simulink model "SDT_Control_Tuning"  (R2025b)
settings: Solver=VariableStepAuto  StartTime=0.0  StopTime=10.0  RelTol=1e-3
undefined symbols (not defined in the file or in its folder): boom, C_tile_force, C_tile_torque, CoM_variation_x, CoM_variation_y, CoM_variation_z, Container_x, Container_z, InvDyn, InvDynAug, J_B_B, J_C_C, J_P_P, J_T_T, K_tile_force, K_tile_torque, KIN, m_B, m_C, m_P, m_T, robot, Tile_z, unc_freq_boom, ureal, uss
libraries: SDTlibV1 x73, RCTblocks x39
(part 1 of 5)
settings Model: Creator=l.sekules  LastModifiedBy=l.sekules

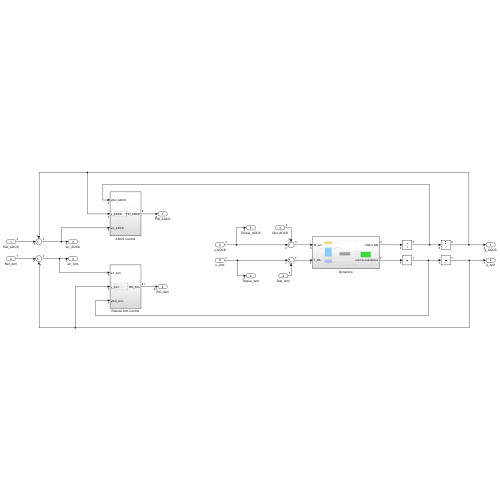
[thumbnail: Simulink's stored preview of the top-level diagram]
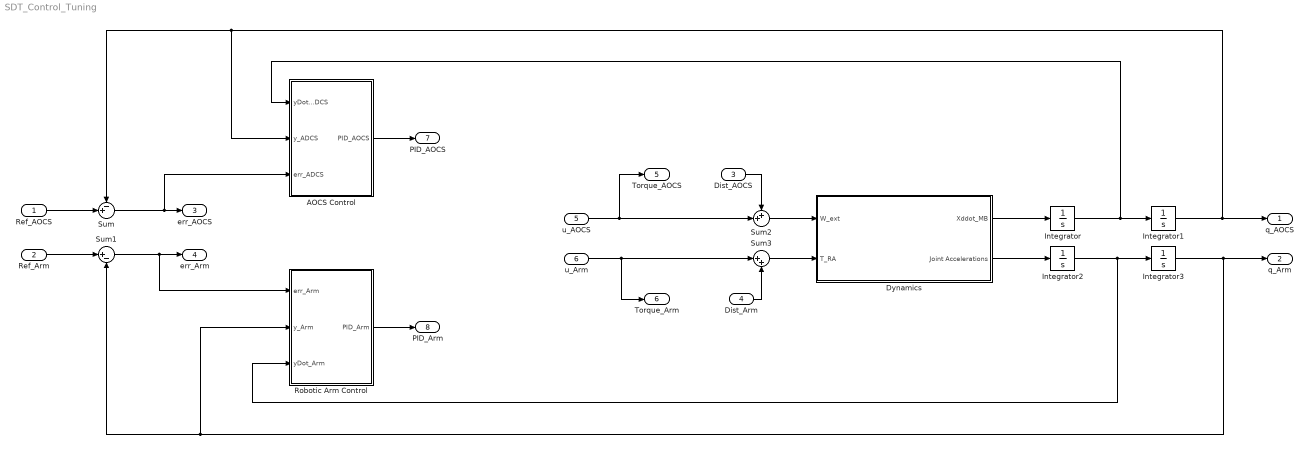
== system SDT_Control_Tuning ==
  Ref_AOCS : Inport  PortDimensions=3
  Ref_Arm : Inport  Port=2  PortDimensions=7
  Dist_AOCS : Inport  Port=3  PortDimensions=3
  Dist_Arm : Inport  Port=4  PortDimensions=7
  u_AOCS : Inport  Port=5  PortDimensions=3
  u_Arm : Inport  Port=6  PortDimensions=7
  AOCS Control : Subsystem
  Dynamics : Subsystem
  Integrator{,1..3} (4 alike) : Integrator
  Robotic Arm Control : Subsystem
  Sum : Sum  Inputs=-+|
  Sum1 : Sum  Inputs=|+-
  Sum2 : Sum  Inputs=++|
  Sum3 : Sum  Inputs=|++
  q_AOCS : Outport
  q_Arm : Outport  Port=2
  err_AOCS : Outport  Port=3
  err_Arm : Outport  Port=4
  Torque_AOCS : Outport  Port=5
  Torque_Arm : Outport  Port=6
  PID_AOCS : Outport  Port=7
  PID_Arm : Outport  Port=8
  wires:
  Integrator1/1 -> AOCS Control/2(y_ADCS), Sum/1, q_AOCS/1
  Integrator3/1 -> Robotic Arm Control/2(y_Arm), Sum1/2, q_Arm/1
  Sum/1 -> AOCS Control/3(err_ADCS), err_AOCS/1
  Sum1/1 -> Robotic Arm Control/1(err_Arm), err_Arm/1
  Ref_AOCS/1 -> Sum/2
  Ref_Arm/1 -> Sum1/1
  Integrator/1 -> AOCS Control/1(yDot_ADCS), Integrator1/1
  Integrator2/1 -> Robotic Arm Control/3(yDot_Arm), Integrator3/1
  AOCS Control/1(PID_AOCS) -> PID_AOCS/1
  Robotic Arm Control/1(PID_Arm) -> PID_Arm/1
  u_Arm/1 -> Torque_Arm/1, Sum3/1
  Dist_Arm/1 -> Sum3/2
  u_AOCS/1 -> Torque_AOCS/1, Sum2/2
  Dist_AOCS/1 -> Sum2/1
  Sum2/1 -> Dynamics/1(W_ext)
  Sum3/1 -> Dynamics/2(T_RA)
  Dynamics/1(Xddot_MB) -> Integrator/1
  Dynamics/2(Joint Accelerations) -> Integrator2/1

== system SDT_Control_Tuning/AOCS Control ==
  yDot_ADCS : Inport
  y_ADCS : Inport  Port=2
  err_ADCS : Inport  Port=3
  Integrator : Integrator
  Mux : Mux  Inputs=3
  PID_AOCS : Outport
  wires:
  err_ADCS/1 -> Integrator/1
  y_ADCS/1 -> Mux/1
  yDot_ADCS/1 -> Mux/3
  Mux/1 -> PID_AOCS/1
  Integrator/1 -> Mux/2

== system SDT_Control_Tuning/Dynamics ==
  W_ext : Inport
  T_RA : Inport  Port=2
  Demux : Demux  Outputs=3
  Demux1 : Demux  Outputs=2
  Flexible Bar : Subsystem
  Ground : Ground
  Main body : Subsystem  mask(Multi-port rigid body (18nx6n)){m=m_B, Ig=J_B_B, OG=[CoM_variation_x;CoM_variation_y;CoM_variation_z], n=4, OP1=[0;0;0], OP2=[0.35;0;2.5], OP3=[0;0;-2.5], OP4=[1.1;0;0.5], OP5=[0;0;0]}
      mask prompts: m "Mass (Kg)"; Ig "Inertia (at G, Kg m^2)"; OG "OG (3x1 vector, m)"; n "Number of ports"; OP1 "OP1 (3x1 vector, m)"; OP2 "OP2 (3x1 vector, m)"; OP3 "OP3 (3x1 vector, m)"; OP4 "OP4 (3x1 vector, m)"; OP5 "OP5 (3x1 vector,m)"
      mask help:
      | 18nx6n dynamic model of a rigid body at n given points (ports) between wrenches applied at the n points (input) and the motions vectors at these points (output).
      |
      | 0: the reference point
      | G: the center of mass
      | Pi (i=1:n): the n given connection points (n<6).
      |
      | All parameters are expressed in the body frame.
      | Each parameter can be an uncertain parameter declared with "ureal"
      mask init:
      | MultiPortRigidFreeBody
      mask Help: web('Docmultiportrigidbase.html','-browser','-browser')
      mask TypeOptions n: 1 | 2 | 3 | 4 | 5
      mask DialogControl ParameterGroupVar Prompt: Main parameters
      mask DialogControl port1 Prompt: Port #1
      mask DialogControl port2 Prompt: #2
      mask DialogControl port3 Prompt: #3
      mask DialogControl port4 Prompt: #4
      mask DialogControl port5 Prompt: #5
      mask Display:
      | disp('Multi-port\n rigid free body\n (18nx6n)')
      | for ii=1:n
      |     port_label('input', ii,['W_{./body,P',num2str(ii),'}'],'interpreter','tex')
      |     port_label('output',ii,['m_{P',num2str(ii),'}'],'interpreter','tex')
      | end
  Multi port rigid body : Subsystem  mask(Multi-port rigid body (18(n-1)+6]x[6(n-1)+18])){m=m_C, Ig=J_C_C, OG=[0;0;0], n=2, numinv=2, OP1=[Container_x/2;0;0], OP2=[0;0;-Container_z/2], OP3=[ureal('P3_y',1,'percent',10);0;0], OP4=[0;0;0], OP5=[0;0;0]}
      mask prompts: m "Mass (Kg)"; Ig "Inertia (at G, Kg m^2)"; OG "OG (3x1 vector, m)"; n "Number of ports"; numinv "The single parent port"; OP1 "OP1 (3x1 vector, m)"; OP2 "OP2 (3x1 vector, m)"; OP3 "OP3 (3x1 vector, m)"; OP4 "OP4 (3x1 vector, m)"; OP5 "OP5 (3x1 vector,m)"
      mask help:
      | [18(n-1)+6]x[6(n-1)+18] dynamic model of a rigid body at n given points (ports) between:
      | * the wrenches applied at the n-1 child ports and  the motion vector at a single parent port (inputs).
      | * the motions vectors at the  n-1 child ports and the wrench applied by the rigid body at the parent port (output)
      |
      | 0: the reference point
      | G: the center of mass
      | Pi (i=1:n): the n given connection points (n<6).
      |
      | All parameters are expressed in the body frame.
      | Each parameter can be an uncertain parameter declared with "ureal"
      |
      | The 6x18 channel associated to the single parent port can be any of the ports.
      mask init:
      | MultiPortRigidBodyAug
      mask Help: web('Docmultiportrigidbody.html','-browser','-browser')
      mask TypeOptions n: 1 | 2 | 3 | 4 | 5
      mask TypeOptions numinv: 1 | 2 | 3 | 4 | 5
      mask DialogControl ParameterGroupVar Prompt: Main parameters
      mask DialogControl port1 Prompt: Port #1
      mask DialogControl port2 Prompt: #2
      mask DialogControl port3 Prompt: #3
      mask DialogControl port4 Prompt: #4
      mask DialogControl port5 Prompt: #5
      mask Display:
      | disp('Multi-port\n rigid body\n [18(n-1)+6]x[6(n-1)+18]')
      | if n==1,
      |     if numinv==1,
      |         port_label('input', 1,'m_P')
      |         port_label('output',1,'Wbody/.,P')
      |     else
      |         port_label('input', 1,'W./body,P')
      |         port_label('output',1,'m_P')
      |     end
      | else
      |     for ii=1:n
      |         if numinv==ii,
      |             port_label('output',ii,['Wbody/.,P',num2str(ii)])
      |             port_label('input', ii,['m_P',num2str(ii)])
      |         else
      |             port_label('input', ii,['W./body,P',num2str(ii)])
      |             port_label('output',ii,['m_P',num2str(ii)])
      |         end
      |     end
      | end
  Mux : Mux  Inputs=2
  Robotic Arm : Subsystem
  Terminator : Terminator
  Terminator1 : Terminator
  Terminator2 : Terminator
  Tiles : Subsystem
  Xddot_MB : Outport
  Joint Accelerations : Outport  Port=2
  wires:
  Main body/4(m_P4) -> Robotic Arm/1(m_P1)
  Robotic Arm/2(Joint Accelerations) -> Joint Accelerations/1
  Demux/3 -> Terminator1/1
  Main body/2(m_P2) -> Multi port rigid body/2(in2)
  Tiles/3(W_EE) -> Robotic Arm/3(W_EE)
  Robotic Arm/1(W_P1) -> Main body/4(W_./body,P4)
  Multi port rigid body/1(out1) -> Tiles/1(m_Container)
  Robotic Arm/3(m_EE) -> Tiles/3(m_EE)
  Flexible Bar/2(m_Endpoint) -> Tiles/2(m_Endpoint)
  Tiles/2(W_Endpoint) -> Flexible Bar/2(W_Endpoint)
  Multi port rigid body/2(out2) -> Main body/2(W_./body,P2)
  Flexible Bar/1(W_body,P3) -> Main body/3(W_./body,P3)
  Main body/3(m_P3) -> Flexible Bar/1(m_P3)
  Main body/1(m_P1) -> Demux/1
  Demux/2 -> Terminator/1
  Tiles/1(W_Container) -> Multi port rigid body/1(in1)
  T_RA/1 -> Robotic Arm/2(T_RA)
  Demux/1 -> Demux1/1
  Demux1/2 -> Xddot_MB/1
  Demux1/1 -> Terminator2/1
  Mux/1 -> Main body/1(W_./body,P1)
  W_ext/1 -> Mux/2
  Ground/1 -> Mux/1

== system SDT_Control_Tuning/Robotic Arm Control ==
  err_Arm : Inport
  y_Arm : Inport  Port=2
  yDot_Arm : Inport  Port=3
  Integrator : Integrator
  Mux : Mux  Inputs=3
  PID_Arm : Outport
  wires:
  yDot_Arm/1 -> Mux/3
  y_Arm/1 -> Mux/1
  Integrator/1 -> Mux/2
  err_Arm/1 -> Integrator/1
  Mux/1 -> PID_Arm/1

== system SDT_Control_Tuning/Dynamics/Flexible Bar ==
  m_P3 : Inport
  W_Endpoint : Inport  Port=2
  " N ports Nastran (free) body" : Subsystem  mask(NINOP Model of a Nastran body){fbdf='boom', ff06='boom', P_gp=1, C_gp=11, nf=boom.n_modes, Xi=boom.damping_ratio, free=off, uw_var=unc_freq_boom, Nflex_w=boom.n_unc, uls_var=0, Nflex_LP=0, uev_var=0, Nflex_EV=0}
      mask prompts: fbdf "Name of the .bdf file (without extension)"; ff06 "Name of the .f06 file (without extension)"; P_gp "Node number corresponding to the point P (connection with parent body)"; C_gp "Node numbers corresponding to the points C (connections with child bodies)"; nf "Number of modes to be considered"; Xi "Common damping ratio"; free "Free body at P"; uw_var "uncertainties (%)"; Nflex_w "number of flexible modes (integer)"; uls_var "uncertainties (%)"; Nflex_LP "number of flexible modes (integer)"; uev_var "uncertainties (%)"; Nflex_EV "number of flexible modes (integer)"
      mask help:
      | NINOP (18n+6)x(6n+18) model of a flexible body at points C (connection point with the child  bodies) and point P (connection point with a parent body).
      | * 18nx6n transfer between the wrench applied to this body at the child points C  and motion vectors at these points
      | * 6x18 transfer between the motion vector at the "parent" point P  and the wrench applied by this body at this point
      | The model is expressed In the (inherit) body frame.
      |
      | Model is built from  the data provided by Patran/Nastran analysis output files.
      | Uncertainties can be added to the main parameters.
      |
      | RK: The last channel associated to parent port P can be inverted to free the body at the point P. In that case, 6 rigid modes (12 integrators) are added in the model to output the motion vector at the point P and the model becomes 18(n+1)x6(n+1).
      mask init:
      | n = length(C_gp);
      | NastranBodyNPortAugFree
      mask Help: web('DocNPortNastranBody.html','-browser','-browser')
      mask DialogControl Container2 Prompt: Main parameters
      mask DialogControl Container6 Prompt: Parametric uncertainties:
      mask DialogControl Container8 Prompt: Frequencies
      mask DialogControl Control18 Prompt: A common relative uncertainty (%) on the first flexible mode frequencies can be added (uncertainties can be changed later)
      mask DialogControl Control3 Prompt: The uncertain frequency is named: 'w_name_i' where:
      mask DialogControl Control4 Prompt: * 'name' is the current block name (reduced to its alphanumeric characters).
      mask DialogControl Control17 Prompt: * 'i' is the flexible mode number (increasing frequency order)
      mask DialogControl Container9 Prompt: Modal participation factors
      mask DialogControl Control20 Prompt: A common relative uncertainty (%) on the modal participation factors of the first flexible modes can be added (uncertainties can be changed later)
      mask DialogControl Control6 Prompt: The uncertain modal participation factor is named: 'LP_name_iXX' where:
      mask DialogControl Control7 Prompt: *  'name' is the current block name (reduced to its alphanumeric characters),
      mask DialogControl Control8 Prompt: * 'i' is the flexible mode number (increasing frequency order),
      mask DialogControl Control9 Prompt: * 'XX' = 'Tx', 'Ty', 'Tz', 'Rx', 'Ry', 'Rz'.
      mask DialogControl Container10 Prompt: Modal shapes
      mask DialogControl Control21 Prompt: A common relative uncertainty (%) on each eigen vector components at points C for the first flexible modes can be added (uncertainties can be changed later)
      mask DialogControl Control16 Prompt: WARNING: can generate very long process time !!
      mask DialogControl Control11 Prompt: The uncertain component is named: "EV_name_Cj_iXX' where:
      mask DialogControl Control12 Prompt: * 'name' is the current block name (reduced to its alphanumeric characters).
      mask DialogControl Control13 Prompt: * 'j' is the point C number,
      mask DialogControl Control14 Prompt: * 'i' is the flexible mode number (increasing frequency order),
      mask DialogControl Control15 Prompt: * 'XX' = 'Tx', 'Ty', 'Tz', 'Rx', 'Ry', 'Rz'.
      mask Display:
      | if free
      |     disp('NINOP (free)\n Nastran body\n 18(n+1)x6(n+1)')
      | else
      |     disp('NINOP (free)\n Nastran body\n (18n+6)x(6n+18)')
      | end
      | 
      | for ii=1:n
      |         port_label('input', ii,['W./body,C',num2str(ii)])
      |         port_label('output',ii,['m_C',num2str(ii)])
      | end
      | 
      | if free
      |     port_label('input', n+1,'W./body,P')
      |     port_label('output',n+1,'m_P')
      | else
      |     port_label('input', n+1,'m_P')
      |     port_label('output',n+1,'Wbody/.,P')
      | end
  18x18 DCM : SDTlibV1/3//6//18 DCM/18x18 DCM  rot=[0 0 1;0 1 0; -1 0 0]'  transp=off
      settings: SourceProductName=SDTlib
  18x18 DCM1 : SDTlibV1/3//6//18 DCM/18x18 DCM  rot=[0 -1 0; 1 0 0; 0 0 1]'  transp=off
      settings: SourceProductName=SDTlib
  18x18 DCM2 : SDTlibV1/3//6//18 DCM/18x18 DCM  rot=[0 0 1;0 1 0; -1 0 0]  transp=off
      settings: SourceProductName=SDTlib
  6x6 DCM : SDTlibV1/3//6//18 DCM/6x6 DCM  rot=[0 0 1;0 1 0; -1 0 0]  transp=off
      settings: SourceProductName=SDTlib
  6x6 DCM1 : SDTlibV1/3//6//18 DCM/6x6 DCM  rot=[0 -1 0; 1 0 0; 0 0 1]  transp=off
      settings: SourceProductName=SDTlib
  6x6 DCM2 : SDTlibV1/3//6//18 DCM/6x6 DCM  rot=[0 0 1;0 1 0; -1 0 0]'  transp=off
      settings: SourceProductName=SDTlib
  Multi port rigid body1 : Subsystem  mask(Multi-port rigid body (18(n-1)+6]x[6(n-1)+18])){m=m_P, Ig=J_P_P, OG=[0;0;0], n=2, numinv=1, OP1=[0;0;0.2], OP2=[0.1;0;-0.1], OP3=[ureal('P3_y',1,'percent',10);0;0], OP4=[0;0;0], OP5=[0;0;0]}
      mask prompts: m "Mass (Kg)"; Ig "Inertia (at G, Kg m^2)"; OG "OG (3x1 vector, m)"; n "Number of ports"; numinv "The single parent port"; OP1 "OP1 (3x1 vector, m)"; OP2 "OP2 (3x1 vector, m)"; OP3 "OP3 (3x1 vector, m)"; OP4 "OP4 (3x1 vector, m)"; OP5 "OP5 (3x1 vector,m)"
      mask help:
      | [18(n-1)+6]x[6(n-1)+18] dynamic model of a rigid body at n given points (ports) between:
      | * the wrenches applied at the n-1 child ports and  the motion vector at a single parent port (inputs).
      | * the motions vectors at the  n-1 child ports and the wrench applied by the rigid body at the parent port (output)
      |
      | 0: the reference point
      | G: the center of mass
      | Pi (i=1:n): the n given connection points (n<6).
      |
      | All parameters are expressed in the body frame.
      | Each parameter can be an uncertain parameter declared with "ureal"
      |
      | The 6x18 channel associated to the single parent port can be any of the ports.
      mask init:
      | MultiPortRigidBodyAug
      mask Help: web('Docmultiportrigidbody.html','-browser','-browser')
      mask TypeOptions n: 1 | 2 | 3 | 4 | 5
      mask TypeOptions numinv: 1 | 2 | 3 | 4 | 5
      mask DialogControl ParameterGroupVar Prompt: Main parameters
      mask DialogControl port1 Prompt: Port #1
      mask DialogControl port2 Prompt: #2
      mask DialogControl port3 Prompt: #3
      mask DialogControl port4 Prompt: #4
      mask DialogControl port5 Prompt: #5
      mask Display:
      | disp('Multi-port\n rigid body\n [18(n-1)+6]x[6(n-1)+18]')
      | if n==1,
      |     if numinv==1,
      |         port_label('input', 1,'m_P')
      |         port_label('output',1,'Wbody/.,P')
      |     else
      |         port_label('input', 1,'W./body,P')
      |         port_label('output',1,'m_P')
      |     end
      | else
      |     for ii=1:n
      |         if numinv==ii,
      |             port_label('output',ii,['Wbody/.,P',num2str(ii)])
      |             port_label('input', ii,['m_P',num2str(ii)])
      |         else
      |             port_label('input', ii,['W./body,P',num2str(ii)])
      |             port_label('output',ii,['m_P',num2str(ii)])
      |         end
      |     end
      | end
  Multi port rigid body2 : Subsystem  mask(Multi-port rigid body (18(n-1)+6]x[6(n-1)+18])){m=m_P, Ig=J_P_P, OG=[0;0;0], n=2, numinv=1, OP1=[-0.1 0 -0.1], OP2=[0 0 0.2], OP3=[ureal('P3_y',1,'percent',10);0;0], OP4=[0;0;0], OP5=[0;0;0]}
      mask prompts: m "Mass (Kg)"; Ig "Inertia (at G, Kg m^2)"; OG "OG (3x1 vector, m)"; n "Number of ports"; numinv "The single parent port"; OP1 "OP1 (3x1 vector, m)"; OP2 "OP2 (3x1 vector, m)"; OP3 "OP3 (3x1 vector, m)"; OP4 "OP4 (3x1 vector, m)"; OP5 "OP5 (3x1 vector,m)"
      mask help:
      | [18(n-1)+6]x[6(n-1)+18] dynamic model of a rigid body at n given points (ports) between:
      | * the wrenches applied at the n-1 child ports and  the motion vector at a single parent port (inputs).
      | * the motions vectors at the  n-1 child ports and the wrench applied by the rigid body at the parent port (output)
      |
      | 0: the reference point
      | G: the center of mass
      | Pi (i=1:n): the n given connection points (n<6).
      |
      | All parameters are expressed in the body frame.
      | Each parameter can be an uncertain parameter declared with "ureal"
      |
      | The 6x18 channel associated to the single parent port can be any of the ports.
      mask init:
      | MultiPortRigidBodyAug
      mask Help: web('Docmultiportrigidbody.html','-browser','-browser')
      mask TypeOptions n: 1 | 2 | 3 | 4 | 5
      mask TypeOptions numinv: 1 | 2 | 3 | 4 | 5
      mask DialogControl ParameterGroupVar Prompt: Main parameters
      mask DialogControl port1 Prompt: Port #1
      mask DialogControl port2 Prompt: #2
      mask DialogControl port3 Prompt: #3
      mask DialogControl port4 Prompt: #4
      mask DialogControl port5 Prompt: #5
      mask Display:
      | disp('Multi-port\n rigid body\n [18(n-1)+6]x[6(n-1)+18]')
      | if n==1,
      |     if numinv==1,
      |         port_label('input', 1,'m_P')
      |         port_label('output',1,'Wbody/.,P')
      |     else
      |         port_label('input', 1,'W./body,P')
      |         port_label('output',1,'m_P')
      |     end
      | else
      |     for ii=1:n
      |         if numinv==ii,
      |             port_label('output',ii,['Wbody/.,P',num2str(ii)])
      |             port_label('input', ii,['m_P',num2str(ii)])
      |         else
      |             port_label('input', ii,['W./body,P',num2str(ii)])
      |             port_label('output',ii,['m_P',num2str(ii)])
      |         end
      |     end
      | end
  W_body,P3 : Outport
  m_Endpoint : Outport  Port=2
  wires:
  " N ports Nastran (free) body"/2(out2) -> 6x6 DCM/1
  " N ports Nastran (free) body"/1(out1) -> 18x18 DCM2/1
  Multi port rigid body1/2(out2) -> 18x18 DCM/1
  6x6 DCM2/1 -> " N ports Nastran (free) body"/1(in1)
  18x18 DCM2/1 -> Multi port rigid body2/1(in1)
  6x6 DCM/1 -> Multi port rigid body1/2(in2)
  18x18 DCM/1 -> " N ports Nastran (free) body"/2(in2)
  Multi port rigid body2/1(out1) -> 6x6 DCM2/1
  6x6 DCM1/1 -> Multi port rigid body2/2(in2)
  Multi port rigid body2/2(out2) -> 18x18 DCM1/1
  Multi port rigid body1/1(out1) -> W_body,P3/1
  m_P3/1 -> Multi port rigid body1/1(in1)
  18x18 DCM1/1 -> m_Endpoint/1
  W_Endpoint/1 -> 6x6 DCM1/1

== system SDT_Control_Tuning/Dynamics/Main body ==
  W_./body,P1 : Inport  PortDimensions=6
  W_./body,P2 : Inport  Port=2  PortDimensions=6
  W_./body,P3 : Inport  Port=3  PortDimensions=6
  W_./body,P4 : Inport  Port=4  PortDimensions=6
  Demux : Demux  Outputs=[18 18 18 18]
  Gain : RCTblocks/Uncertain State Space  Tag=USS  USystem=uss(InvDyn)  UValue=[]  X0=[]  uX0=[]
  Mux : Mux  Inputs=[6 6 6 6]
  m_P1 : Outport
  m_P2 : Outport  Port=2
  m_P3 : Outport  Port=3
  m_P4 : Outport  Port=4
  wires:
  Mux/1 -> Gain/1
  Gain/1 -> Demux/1
  W_./body,P1/1 -> Mux/1
  Demux/1 -> m_P1/1
  W_./body,P2/1 -> Mux/2
  Demux/2 -> m_P2/1
  W_./body,P3/1 -> Mux/3
  Demux/3 -> m_P3/1
  W_./body,P4/1 -> Mux/4
  Demux/4 -> m_P4/1

== system SDT_Control_Tuning/Dynamics/Multi port rigid body ==
  in1 : Inport  PortDimensions=6
  in2 : Inport  Port=2  PortDimensions=18
  Demux : Demux  Outputs=[ 18 6]
  Gain : RCTblocks/Uncertain State Space  Tag=USS  USystem=uss(InvDynAug)  UValue=[]  X0=[]  uX0=[]
  Mux : Mux  Inputs=[ 6 18]
  out1 : Outport
  out2 : Outport  Port=2
  wires:
  Mux/1 -> Gain/1
  Gain/1 -> Demux/1
  in1/1 -> Mux/1
  Demux/1 -> out1/1
  in2/1 -> Mux/2
  Demux/2 -> out2/1

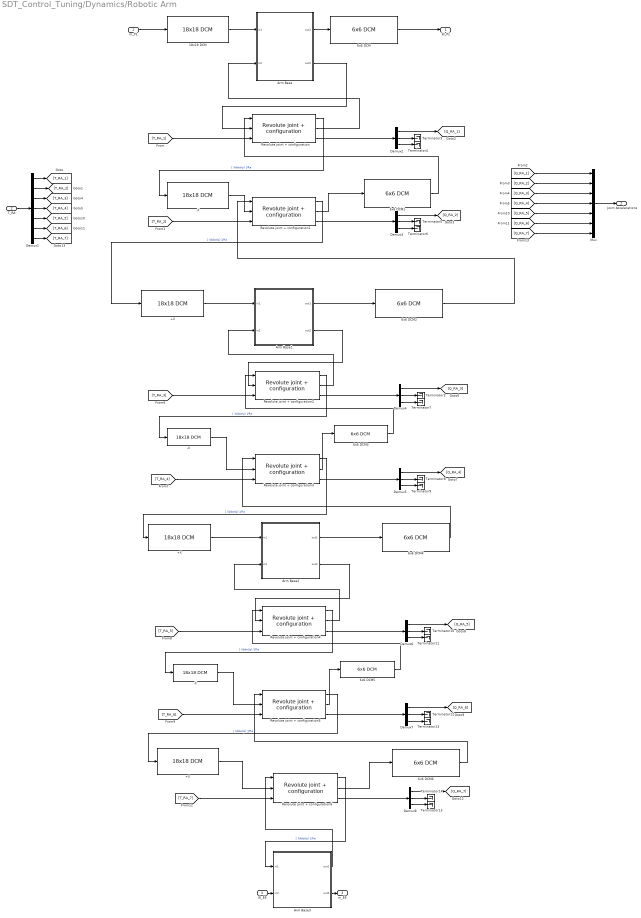
== system SDT_Control_Tuning/Dynamics/Robotic Arm ==
  m_P1 : Inport
  T_RA : Inport  Port=2
  W_EE : Inport  Port=3
  +X : SDTlibV1/3//6//18 DCM/18x18 DCM  rot=[1 0 0; 0 0 1; 0 -1 0]  transp=off
      settings: SourceProductName=SDTlib
  "+X " : SDTlibV1/3//6//18 DCM/18x18 DCM  rot=[1 0 0; 0 0 1; 0 -1 0]  transp=off
      settings: SourceProductName=SDTlib
  "+X  " : SDTlibV1/3//6//18 DCM/18x18 DCM  rot=[1 0 0; 0 0 1; 0 -1 0]  transp=off
      settings: SourceProductName=SDTlib
  -X : SDTlibV1/3//6//18 DCM/18x18 DCM  rot=[1 0 0; 0 0 1; 0 -1 0]  transp=on
      settings: SourceProductName=SDTlib
  "-X " : SDTlibV1/3//6//18 DCM/18x18 DCM  rot=[1 0 0; 0 0 1; 0 -1 0]  transp=on
      settings: SourceProductName=SDTlib
  "-X   " : SDTlibV1/3//6//18 DCM/18x18 DCM  rot=[1 0 0; 0 0 1; 0 -1 0]  transp=on
      settings: SourceProductName=SDTlib
  18x18 DCM : SDTlibV1/3//6//18 DCM/18x18 DCM  rot=[0 0 1;0 1 0; -1 0 0]'  transp=off
      settings: SourceProductName=SDTlib
  6x6 DCM : SDTlibV1/3//6//18 DCM/6x6 DCM  rot=[0 0 1;0 1 0; -1 0 0]  transp=off
      settings: SourceProductName=SDTlib
  6x6 DCM1 : SDTlibV1/3//6//18 DCM/6x6 DCM  rot=[1 0 0; 0 0 1; 0 -1 0]  transp=off
      settings: SourceProductName=SDTlib
  6x6 DCM2 : SDTlibV1/3//6//18 DCM/6x6 DCM  rot=[1 0 0; 0 0 1; 0 -1 0]  transp=on
      settings: SourceProductName=SDTlib
  6x6 DCM3 : SDTlibV1/3//6//18 DCM/6x6 DCM  rot=[1 0 0; 0 0 1; 0 -1 0]  transp=off
      settings: SourceProductName=SDTlib
  6x6 DCM4 : SDTlibV1/3//6//18 DCM/6x6 DCM  rot=[1 0 0; 0 0 1; 0 -1 0]  transp=on
      settings: SourceProductName=SDTlib
  6x6 DCM5 : SDTlibV1/3//6//18 DCM/6x6 DCM  rot=[1 0 0; 0 0 1; 0 -1 0]  transp=off
      settings: SourceProductName=SDTlib
  6x6 DCM6 : SDTlibV1/3//6//18 DCM/6x6 DCM  rot=[1 0 0; 0 0 1; 0 -1 0]  transp=on
      settings: SourceProductName=SDTlib
  Arm Base : Subsystem  mask(Multi-port rigid body (18(n-1)+6]x[6(n-1)+18])){m=robot.linkMass{1,1}, Ig=robot.linkInertia{1,1}, OG=[0;0;0], n=2, numinv=1, OP1=[0;0;-robot.linkLength(1)/2], OP2=[0;0;robot.linkLength(1)/2], OP3=[ureal('P3_y',1,'percent',10);0;0], OP4=[0;0;0], OP5=[0;0;0]}
      mask prompts: m "Mass (Kg)"; Ig "Inertia (at G, Kg m^2)"; OG "OG (3x1 vector, m)"; n "Number of ports"; numinv "The single parent port"; OP1 "OP1 (3x1 vector, m)"; OP2 "OP2 (3x1 vector, m)"; OP3 "OP3 (3x1 vector, m)"; OP4 "OP4 (3x1 vector, m)"; OP5 "OP5 (3x1 vector,m)"
      mask help:
      | [18(n-1)+6]x[6(n-1)+18] dynamic model of a rigid body at n given points (ports) between:
      | * the wrenches applied at the n-1 child ports and  the motion vector at a single parent port (inputs).
      | * the motions vectors at the  n-1 child ports and the wrench applied by the rigid body at the parent port (output)
      |
      | 0: the reference point
      | G: the center of mass
      | Pi (i=1:n): the n given connection points (n<6).
      |
      | All parameters are expressed in the body frame.
      | Each parameter can be an uncertain parameter declared with "ureal"
      |
      | The 6x18 channel associated to the single parent port can be any of the ports.
      mask init:
      | MultiPortRigidBodyAug
      mask Help: web('Docmultiportrigidbody.html','-browser','-browser')
      mask TypeOptions n: 1 | 2 | 3 | 4 | 5
      mask TypeOptions numinv: 1 | 2 | 3 | 4 | 5
      mask DialogControl ParameterGroupVar Prompt: Main parameters
      mask DialogControl port1 Prompt: Port #1
      mask DialogControl port2 Prompt: #2
      mask DialogControl port3 Prompt: #3
      mask DialogControl port4 Prompt: #4
      mask DialogControl port5 Prompt: #5
      mask Display:
      | disp('Multi-port\n rigid body\n [18(n-1)+6]x[6(n-1)+18]')
      | if n==1,
      |     if numinv==1,
      |         port_label('input', 1,'m_P')
      |         port_label('output',1,'Wbody/.,P')
      |     else
      |         port_label('input', 1,'W./body,P')
      |         port_label('output',1,'m_P')
      |     end
      | else
      |     for ii=1:n
      |         if numinv==ii,
      |             port_label('output',ii,['Wbody/.,P',num2str(ii)])
      |             port_label('input', ii,['m_P',num2str(ii)])
      |         else
      |             port_label('input', ii,['W./body,P',num2str(ii)])
      |             port_label('output',ii,['m_P',num2str(ii)])
      |         end
      |     end
      | end
  Arm Base1 : Subsystem  mask(Multi-port rigid body (18(n-1)+6]x[6(n-1)+18])){m=robot.linkMass{1,2}, Ig=robot.linkInertia{1,2}, OG=[0;0;0], n=2, numinv=1, OP1=[0;0;-robot.linkLength(2)/2], OP2=[0;0;robot.linkLength(2)/2], OP3=[ureal('P3_y',1,'percent',10);0;0], OP4=[0;0;0], OP5=[0;0;0]}
      mask prompts: m "Mass (Kg)"; Ig "Inertia (at G, Kg m^2)"; OG "OG (3x1 vector, m)"; n "Number of ports"; numinv "The single parent port"; OP1 "OP1 (3x1 vector, m)"; OP2 "OP2 (3x1 vector, m)"; OP3 "OP3 (3x1 vector, m)"; OP4 "OP4 (3x1 vector, m)"; OP5 "OP5 (3x1 vector,m)"
      mask help:
      | [18(n-1)+6]x[6(n-1)+18] dynamic model of a rigid body at n given points (ports) between:
      | * the wrenches applied at the n-1 child ports and  the motion vector at a single parent port (inputs).
      | * the motions vectors at the  n-1 child ports and the wrench applied by the rigid body at the parent port (output)
      |
      | 0: the reference point
      | G: the center of mass
      | Pi (i=1:n): the n given connection points (n<6).
      |
      | All parameters are expressed in the body frame.
      | Each parameter can be an uncertain parameter declared with "ureal"
      |
      | The 6x18 channel associated to the single parent port can be any of the ports.
      mask init:
      | MultiPortRigidBodyAug
      mask Help: web('Docmultiportrigidbody.html','-browser','-browser')
      mask TypeOptions n: 1 | 2 | 3 | 4 | 5
      mask TypeOptions numinv: 1 | 2 | 3 | 4 | 5
      mask DialogControl ParameterGroupVar Prompt: Main parameters
      mask DialogControl port1 Prompt: Port #1
      mask DialogControl port2 Prompt: #2
      mask DialogControl port3 Prompt: #3
      mask DialogControl port4 Prompt: #4
      mask DialogControl port5 Prompt: #5
      mask Display:
      | disp('Multi-port\n rigid body\n [18(n-1)+6]x[6(n-1)+18]')
      | if n==1,
      |     if numinv==1,
      |         port_label('input', 1,'m_P')
      |         port_label('output',1,'Wbody/.,P')
      |     else
      |         port_label('input', 1,'W./body,P')
      |         port_label('output',1,'m_P')
      |     end
      | else
      |     for ii=1:n
      |         if numinv==ii,
      |             port_label('output',ii,['Wbody/.,P',num2str(ii)])
      |             port_label('input', ii,['m_P',num2str(ii)])
      |         else
      |             port_label('input', ii,['W./body,P',num2str(ii)])
      |             port_label('output',ii,['m_P',num2str(ii)])
      |         end
      |     end
      | end
  Arm Base2 : Subsystem  mask(Multi-port rigid body (18(n-1)+6]x[6(n-1)+18])){m=robot.linkMass{1,3}, Ig=robot.linkInertia{1,3}, OG=[0;0;0], n=2, numinv=1, OP1=[0;0;-robot.linkLength(3)/2], OP2=[0;0;robot.linkLength(3)/2], OP3=[ureal('P3_y',1,'percent',10);0;0], OP4=[0;0;0], OP5=[0;0;0]}
      mask prompts: m "Mass (Kg)"; Ig "Inertia (at G, Kg m^2)"; OG "OG (3x1 vector, m)"; n "Number of ports"; numinv "The single parent port"; OP1 "OP1 (3x1 vector, m)"; OP2 "OP2 (3x1 vector, m)"; OP3 "OP3 (3x1 vector, m)"; OP4 "OP4 (3x1 vector, m)"; OP5 "OP5 (3x1 vector,m)"
      mask help:
      | [18(n-1)+6]x[6(n-1)+18] dynamic model of a rigid body at n given points (ports) between:
      | * the wrenches applied at the n-1 child ports and  the motion vector at a single parent port (inputs).
      | * the motions vectors at the  n-1 child ports and the wrench applied by the rigid body at the parent port (output)
      |
      | 0: the reference point
      | G: the center of mass
      | Pi (i=1:n): the n given connection points (n<6).
      |
      | All parameters are expressed in the body frame.
      | Each parameter can be an uncertain parameter declared with "ureal"
      |
      | The 6x18 channel associated to the single parent port can be any of the ports.
      mask init:
      | MultiPortRigidBodyAug
      mask Help: web('Docmultiportrigidbody.html','-browser','-browser')
      mask TypeOptions n: 1 | 2 | 3 | 4 | 5
      mask TypeOptions numinv: 1 | 2 | 3 | 4 | 5
      mask DialogControl ParameterGroupVar Prompt: Main parameters
      mask DialogControl port1 Prompt: Port #1
      mask DialogControl port2 Prompt: #2
      mask DialogControl port3 Prompt: #3
      mask DialogControl port4 Prompt: #4
      mask DialogControl port5 Prompt: #5
      mask Display:
      | disp('Multi-port\n rigid body\n [18(n-1)+6]x[6(n-1)+18]')
      | if n==1,
      |     if numinv==1,
      |         port_label('input', 1,'m_P')
      |         port_label('output',1,'Wbody/.,P')
      |     else
      |         port_label('input', 1,'W./body,P')
      |         port_label('output',1,'m_P')
      |     end
      | else
      |     for ii=1:n
      |         if numinv==ii,
      |             port_label('output',ii,['Wbody/.,P',num2str(ii)])
      |             port_label('input', ii,['m_P',num2str(ii)])
      |         else
      |             port_label('input', ii,['W./body,P',num2str(ii)])
      |             port_label('output',ii,['m_P',num2str(ii)])
      |         end
      |     end
      | end
  Arm Base3 : Subsystem  mask(Multi-port rigid body (18(n-1)+6]x[6(n-1)+18])){m=robot.linkMass{1,4}, Ig=robot.linkInertia{1,4}, OG=[0;0;0], n=2, numinv=1, OP1=[0;0;-robot.linkLength(4)/2], OP2=[0;0;robot.linkLength(4)/2], OP3=[ureal('P3_y',1,'percent',10);0;0], OP4=[0;0;0], OP5=[0;0;0]}
      mask prompts: m "Mass (Kg)"; Ig "Inertia (at G, Kg m^2)"; OG "OG (3x1 vector, m)"; n "Number of ports"; numinv "The single parent port"; OP1 "OP1 (3x1 vector, m)"; OP2 "OP2 (3x1 vector, m)"; OP3 "OP3 (3x1 vector, m)"; OP4 "OP4 (3x1 vector, m)"; OP5 "OP5 (3x1 vector,m)"
      mask help:
      | [18(n-1)+6]x[6(n-1)+18] dynamic model of a rigid body at n given points (ports) between:
      | * the wrenches applied at the n-1 child ports and  the motion vector at a single parent port (inputs).
      | * the motions vectors at the  n-1 child ports and the wrench applied by the rigid body at the parent port (output)
      |
      | 0: the reference point
      | G: the center of mass
      | Pi (i=1:n): the n given connection points (n<6).
      |
      | All parameters are expressed in the body frame.
      | Each parameter can be an uncertain parameter declared with "ureal"
      |
      | The 6x18 channel associated to the single parent port can be any of the ports.
      mask init:
      | MultiPortRigidBodyAug
      mask Help: web('Docmultiportrigidbody.html','-browser','-browser')
      mask TypeOptions n: 1 | 2 | 3 | 4 | 5
      mask TypeOptions numinv: 1 | 2 | 3 | 4 | 5
      mask DialogControl ParameterGroupVar Prompt: Main parameters
      mask DialogControl port1 Prompt: Port #1
      mask DialogControl port2 Prompt: #2
      mask DialogControl port3 Prompt: #3
      mask DialogControl port4 Prompt: #4
      mask DialogControl port5 Prompt: #5
      mask Display:
      | disp('Multi-port\n rigid body\n [18(n-1)+6]x[6(n-1)+18]')
      | if n==1,
      |     if numinv==1,
      |         port_label('input', 1,'m_P')
      |         port_label('output',1,'Wbody/.,P')
      |     else
      |         port_label('input', 1,'W./body,P')
      |         port_label('output',1,'m_P')
      |     end
      | else
      |     for ii=1:n
      |         if numinv==ii,
      |             port_label('output',ii,['Wbody/.,P',num2str(ii)])
      |             port_label('input', ii,['m_P',num2str(ii)])
      |         else
      |             port_label('input', ii,['W./body,P',num2str(ii)])
      |             port_label('output',ii,['m_P',num2str(ii)])
      |         end
      |     end
      | end
  Demux1 : Demux  Outputs=7
  Demux{2..8} (7 alike) : Demux  Outputs=3
  Mux : Mux  Inputs=7
  Revolute joint + configuration : SDTlibV1/6 dof mechanisms/Revolute joint + configuration  ra=[0;0;1]  Jr=1  theta=robot.config{1}
      settings: SourceProductName=SDTlib
  Revolute joint + configuration1 : SDTlibV1/6 dof mechanisms/Revolute joint + configuration  ra=[0;0;1]  Jr=1  theta=robot.config{2}
      settings: SourceProductName=SDTlib
  Revolute joint + configuration2 : SDTlibV1/6 dof mechanisms/Revolute joint + configuration  ra=[0;0;1]  Jr=1  theta=robot.config{3}
      settings: SourceProductName=SDTlib
  Revolute joint + configuration3 : SDTlibV1/6 dof mechanisms/Revolute joint + configuration  ra=[0;0;1]  Jr=1  theta=robot.config{4}
      settings: SourceProductName=SDTlib
  Revolute joint + configuration4 : SDTlibV1/6 dof mechanisms/Revolute joint + configuration  ra=[0;0;1]  Jr=1  theta=robot.config{5}
      settings: SourceProductName=SDTlib
  Revolute joint + configuration5 : SDTlibV1/6 dof mechanisms/Revolute joint + configuration  ra=[0;0;1]  Jr=1  theta=robot.config{6}
      settings: SourceProductName=SDTlib
  Revolute joint + configuration6 : SDTlibV1/6 dof mechanisms/Revolute joint + configuration  ra=[0;0;1]  Jr=1  theta=robot.config{7}
      settings: SourceProductName=SDTlib
  Terminator{2..15} (14 alike) : Terminator
  W_P1 : Outport
  Joint Accelerations : Outport  Port=2
  m_EE : Outport  Port=3
  wires:
  Demux4/3 -> Terminator7/1
  6x6 DCM3/1 -> Revolute joint + configuration2/1
  Demux6/1 -> [Q_RA_5]
  Demux8/1 -> [Q_RA_7]
  [Q_RA_3] -> Mux/3
  Demux7/2 -> Terminator12/1
  Revolute joint + configuration/2 -> Arm Base/2(in2)
  Demux3/1 -> [Q_RA_2]
  [T_RA_3] -> Revolute joint + configuration2/3
  Arm Base/1(out1) -> 6x6 DCM/1
  Revolute joint + configuration4/2 -> Arm Base2/2(in2)
  Arm Base3/1(out1) -> Revolute joint + configuration6/1
  Revolute joint + configuration/1 -> "-X "/1  "[ Xddot(p) ]/Ra"
  [T_RA_7] -> Revolute joint + configuration6/3
  Arm Base/2(out2) -> Revolute joint + configuration/2
  [T_RA_4] -> Revolute joint + configuration3/3
  Revolute joint + configuration5/3 -> Demux7/1
  Demux8/2 -> Terminator14/1
  Revolute joint + configuration4/3 -> Demux6/1
  Demux2/2 -> Terminator3/1
  [T_RA_5] -> Revolute joint + configuration4/3
  "+X  "/1 -> Revolute joint + configuration6/2
  [T_RA_1] -> Revolute joint + configuration/3
  Demux7/3 -> Terminator13/1
  Demux3/2 -> Terminator5/1
  Demux1/4 -> [T_RA_4]
  Revolute joint + configuration2/1 -> -X/1  "[ Xddot(p) ]/Ra"
  W_EE/1 -> Arm Base3/2(in2)
  Arm Base1/2(out2) -> Revolute joint + configuration2/2
  T_RA/1 -> Demux1/1
  Revolute joint + configuration2/3 -> Demux4/1
  Revolute joint + configuration/3 -> Demux2/1
  Demux7/1 -> [Q_RA_6]
  [Q_RA_4] -> Mux/4
  Demux1/2 -> [T_RA_2]
  Demux1/3 -> [T_RA_3]
  Demux6/2 -> Terminator10/1
  Demux6/3 -> Terminator11/1
  [Q_RA_5] -> Mux/5
  18x18 DCM/1 -> Arm Base/1(in1)
  "-X   "/1 -> Revolute joint + configuration5/2
  "-X "/1 -> Revolute joint + configuration1/2
  Demux3/3 -> Terminator6/1
  6x6 DCM5/1 -> Revolute joint + configuration4/1
  Arm Base2/1(out1) -> 6x6 DCM4/1
  Demux2/3 -> Terminator4/1
  Revolute joint + configuration4/1 -> "-X   "/1  "[ Xddot(p) ]/Ra"
  Revolute joint + configuration6/1 -> Arm Base3/1(in1)  "[ Xddot(p) ]/Ra"
  Demux4/2 -> Terminator2/1
  Revolute joint + configuration1/2 -> 6x6 DCM1/1
  [T_RA_6] -> Revolute joint + configuration5/3
  Revolute joint + configuration3/1 -> "+X "/1  "[ Xddot(p) ]/Ra"
  Demux5/1 -> [Q_RA_4]
  [T_RA_2] -> Revolute joint + configuration1/3
  [Q_RA_2] -> Mux/2
  "+X "/1 -> Arm Base2/1(in1)
  Mux/1 -> Joint Accelerations/1
  Demux4/1 -> [Q_RA_3]
  6x6 DCM1/1 -> Revolute joint + configuration/1
  Demux5/2 -> Terminator8/1
  +X/1 -> Arm Base1/1(in1)
  Revolute joint + configuration1/3 -> Demux3/1
  Revolute joint + configuration3/2 -> 6x6 DCM3/1
  -X/1 -> Revolute joint + configuration3/2
  Revolute joint + configuration2/2 -> Arm Base1/2(in2)
  6x6 DCM6/1 -> Revolute joint + configuration5/1
  Demux2/1 -> [Q_RA_1]
  Revolute joint + configuration6/3 -> Demux8/1
  Demux5/3 -> Terminator9/1
  [Q_RA_7] -> Mux/7
  [Q_RA_6] -> Mux/6
  Arm Base1/1(out1) -> 6x6 DCM2/1
  6x6 DCM4/1 -> Revolute joint + configuration3/1
  [Q_RA_1] -> Mux/1
  Revolute joint + configuration1/1 -> +X/1  "[ Xddot(p) ]/Ra"
  Revolute joint + configuration3/3 -> Demux5/1
  6x6 DCM2/1 -> Revolute joint + configuration1/1
  Demux1/1 -> [T_RA_1]
  Demux8/3 -> Terminator15/1
  Revolute joint + configuration6/2 -> 6x6 DCM6/1
  Arm Base2/2(out2) -> Revolute joint + configuration4/2
  Revolute joint + configuration5/2 -> 6x6 DCM5/1
  Revolute joint + configuration5/1 -> "+X  "/1  "[ Xddot(p) ]/Ra"
  Demux1/6 -> [T_RA_6]
  Demux1/5 -> [T_RA_5]
  Demux1/7 -> [T_RA_7]
  m_P1/1 -> 18x18 DCM/1
  6x6 DCM/1 -> W_P1/1
  Arm Base3/2(out2) -> m_EE/1

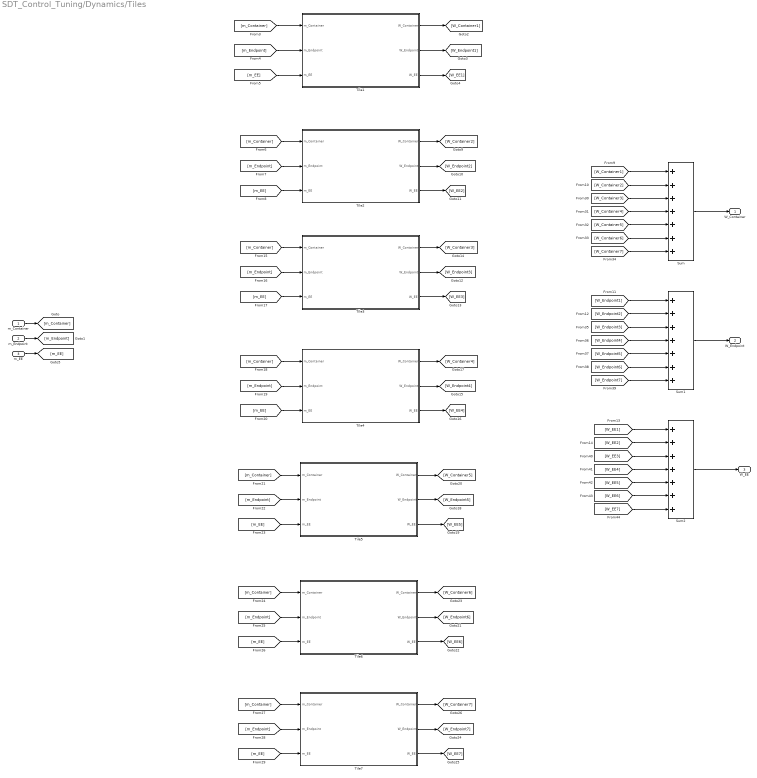
== system SDT_Control_Tuning/Dynamics/Tiles ==
  m_Container : Inport
  m_Endpoint : Inport  Port=2
  m_EE : Inport  Port=3
  Sum : Sum  Inputs=+++++++
  Sum1 : Sum  Inputs=+++++++
  Sum2 : Sum  Inputs=+++++++
  Tile1 : Subsystem
  Tile2 : Subsystem
  Tile3 : Subsystem
  Tile4 : Subsystem
  Tile5 : Subsystem
  Tile6 : Subsystem
  Tile7 : Subsystem
  W_Container : Outport
  W_Endpoint : Outport  Port=2
  W_EE : Outport  Port=3
  wires:
  [m_EE] -> Tile4/3(m_EE)
  [W_EE7] -> Sum2/7
  [m_Endpoint] -> Tile2/2(m_Endpoint)
  [m_Container] -> Tile7/1(m_Container)
  Tile1/2(W_Endpoint) -> [W_Endpoint1]
  [W_EE4] -> Sum2/4
  Sum1/1 -> W_Endpoint/1
  Tile6/3(W_EE) -> [W_EE6]
  Tile4/2(W_Endpoint) -> [W_Endpoint4]
  [m_Endpoint] -> Tile4/2(m_Endpoint)
  [m_EE] -> Tile1/3(m_EE)
  Tile3/3(W_EE) -> [W_EE3]
  [W_Endpoint2] -> Sum1/2
  [W_EE3] -> Sum2/3
  [W_Container3] -> Sum/3
  [m_Container] -> Tile5/1(m_Container)
  [W_Container2] -> Sum/2
  Tile3/1(W_Container) -> [W_Container3]
  [W_Container5] -> Sum/5
  Tile1/3(W_EE) -> [W_EE1]
  [m_EE] -> Tile3/3(m_EE)
  [W_Endpoint6] -> Sum1/6
  [W_EE6] -> Sum2/6
  [W_EE5] -> Sum2/5
  [W_Endpoint5] -> Sum1/5
  [m_EE] -> Tile5/3(m_EE)
  Tile2/3(W_EE) -> [W_EE2]
  [m_EE] -> Tile2/3(m_EE)
  [m_Endpoint] -> Tile7/2(m_Endpoint)
  Tile2/2(W_Endpoint) -> [W_Endpoint2]
  Tile4/1(W_Container) -> [W_Container4]
  [W_Container6] -> Sum/6
  [m_Endpoint] -> Tile3/2(m_Endpoint)
  Tile5/2(W_Endpoint) -> [W_Endpoint5]
  [m_Container] -> Tile1/1(m_Container)
  [W_Endpoint7] -> Sum1/7
  [m_EE] -> Tile6/3(m_EE)
  Tile3/2(W_Endpoint) -> [W_Endpoint3]
  Tile6/1(W_Container) -> [W_Container6]
  [W_Container7] -> Sum/7
  [m_Container] -> Tile3/1(m_Container)
  Tile6/2(W_Endpoint) -> [W_Endpoint6]
  [W_Endpoint1] -> Sum1/1
  [m_Container] -> Tile4/1(m_Container)
  Tile7/2(W_Endpoint) -> [W_Endpoint7]
  Tile5/1(W_Container) -> [W_Container5]
  [W_Container1] -> Sum/1
  [m_Endpoint] -> Tile5/2(m_Endpoint)
  [W_Endpoint3] -> Sum1/3
  [W_Container4] -> Sum/4
  [W_EE1] -> Sum2/1
  Tile1/1(W_Container) -> [W_Container1]
  Tile5/3(W_EE) -> [W_EE5]
  [W_EE2] -> Sum2/2
  [m_Endpoint] -> Tile6/2(m_Endpoint)
  [m_Container] -> Tile2/1(m_Container)
  [m_EE] -> Tile7/3(m_EE)
  [m_Endpoint] -> Tile1/2(m_Endpoint)
  Tile7/1(W_Container) -> [W_Container7]
  [W_Endpoint4] -> Sum1/4
  [m_Container] -> Tile6/1(m_Container)
  Tile4/3(W_EE) -> [W_EE4]
  Tile2/1(W_Container) -> [W_Container2]
  Tile7/3(W_EE) -> [W_EE7]
  Sum/1 -> W_Container/1
  Sum2/1 -> W_EE/1
  m_Container/1 -> [m_Container]
  m_Endpoint/1 -> [m_Endpoint]
  m_EE/1 -> [m_EE]

== system SDT_Control_Tuning/Dynamics/Flexible Bar/ N ports Nastran (free) body ==
  in1 : Inport  PortDimensions=6
  in2 : Inport  Port=2  PortDimensions=18
  Demux : Demux  Outputs=[18 6]
  Gain : RCTblocks/Uncertain State Space  Tag=USS  USystem=Mdyn  UValue=[]  X0=[]  uX0=[]
  Mux : Mux  Inputs=[6 18]
  out1 : Outport
  out2 : Outport  Port=2
  wires:
  Mux/1 -> Gain/1
  Gain/1 -> Demux/1
  in1/1 -> Mux/1
  Demux/1 -> out1/1
  in2/1 -> Mux/2
  Demux/2 -> out2/1

== system SDT_Control_Tuning/Dynamics/Flexible Bar/Multi port rigid body1 ==
  in1 : Inport  PortDimensions=18
  in2 : Inport  Port=2  PortDimensions=6
  Demux : Demux  Outputs=[ 6 18]
  Gain : RCTblocks/Uncertain State Space  Tag=USS  USystem=uss(InvDynAug)  UValue=[]  X0=[]  uX0=[]
  Mux : Mux  Inputs=[ 18 6]
  out1 : Outport
  out2 : Outport  Port=2
  wires:
  Demux/2 -> out2/1
  in2/1 -> Mux/2
  Demux/1 -> out1/1
  in1/1 -> Mux/1
  Gain/1 -> Demux/1
  Mux/1 -> Gain/1

== system SDT_Control_Tuning/Dynamics/Flexible Bar/Multi port rigid body2 ==
  in1 : Inport  PortDimensions=18
  in2 : Inport  Port=2  PortDimensions=6
  Demux : Demux  Outputs=[ 6 18]
  Gain : RCTblocks/Uncertain State Space  Tag=USS  USystem=uss(InvDynAug)  UValue=[]  X0=[]  uX0=[]
  Mux : Mux  Inputs=[ 18 6]
  out1 : Outport
  out2 : Outport  Port=2
  wires:
  Mux/1 -> Gain/1
  Gain/1 -> Demux/1
  in1/1 -> Mux/1
  Demux/1 -> out1/1
  in2/1 -> Mux/2
  Demux/2 -> out2/1

== system SDT_Control_Tuning/Dynamics/Robotic Arm/Arm Base ==
  in1 : Inport  PortDimensions=18
  in2 : Inport  Port=2  PortDimensions=6
  Demux : Demux  Outputs=[ 6 18]
  Gain : RCTblocks/Uncertain State Space  Tag=USS  USystem=uss(InvDynAug)  UValue=[]  X0=[]  uX0=[]
  Mux : Mux  Inputs=[ 18 6]
  out1 : Outport
  out2 : Outport  Port=2
  wires:
  Demux/2 -> out2/1
  in2/1 -> Mux/2
  Demux/1 -> out1/1
  in1/1 -> Mux/1
  Gain/1 -> Demux/1
  Mux/1 -> Gain/1

== system SDT_Control_Tuning/Dynamics/Robotic Arm/Arm Base1 ==
  in1 : Inport  PortDimensions=18
  in2 : Inport  Port=2  PortDimensions=6
  Demux : Demux  Outputs=[ 6 18]
  Gain : RCTblocks/Uncertain State Space  Tag=USS  USystem=uss(InvDynAug)  UValue=[]  X0=[]  uX0=[]
  Mux : Mux  Inputs=[ 18 6]
  out1 : Outport
  out2 : Outport  Port=2
  wires:
  Mux/1 -> Gain/1
  Gain/1 -> Demux/1
  in1/1 -> Mux/1
  Demux/1 -> out1/1
  in2/1 -> Mux/2
  Demux/2 -> out2/1

== system SDT_Control_Tuning/Dynamics/Robotic Arm/Arm Base2 ==
  in1 : Inport  PortDimensions=18
  in2 : Inport  Port=2  PortDimensions=6
  Demux : Demux  Outputs=[ 6 18]
  Gain : RCTblocks/Uncertain State Space  Tag=USS  USystem=uss(InvDynAug)  UValue=[]  X0=[]  uX0=[]
  Mux : Mux  Inputs=[ 18 6]
  out1 : Outport
  out2 : Outport  Port=2
  wires:
  Demux/2 -> out2/1
  in2/1 -> Mux/2
  Demux/1 -> out1/1
  in1/1 -> Mux/1
  Gain/1 -> Demux/1
  Mux/1 -> Gain/1

== system SDT_Control_Tuning/Dynamics/Robotic Arm/Arm Base3 ==
  in1 : Inport  PortDimensions=18
  in2 : Inport  Port=2  PortDimensions=6
  Demux : Demux  Outputs=[ 6 18]
  Gain : RCTblocks/Uncertain State Space  Tag=USS  USystem=uss(InvDynAug)  UValue=[]  X0=[]  uX0=[]
  Mux : Mux  Inputs=[ 18 6]
  out1 : Outport
  out2 : Outport  Port=2
  wires:
  Mux/1 -> Gain/1
  Gain/1 -> Demux/1
  in1/1 -> Mux/1
  Demux/1 -> out1/1
  in2/1 -> Mux/2
  Demux/2 -> out2/1

== system SDT_Control_Tuning/Dynamics/Tiles/Tile1 ==
  m_Container : Inport
  m_Endpoint : Inport  Port=2
  m_EE : Inport  Port=3
  18x18 DCM : SDTlibV1/3//6//18 DCM/18x18 DCM  rot=[0 1 0; 1 0 0; 0 0 -1]  transp=on
      settings: SourceProductName=SDTlib
  6x6 DCM : SDTlibV1/3//6//18 DCM/6x6 DCM  rot=[0 1 0; 1 0 0; 0 0 -1]  transp=off
      settings: SourceProductName=SDTlib
  Depose1 : Subsystem  Commented=on
  Starting Position1 : Subsystem  Commented=on
  Tile : Subsystem  mask(Multi-port rigid body (18nx6n)){m=m_T, Ig=J_T_T, OG=[0;0;0], n=2, OP1=[0;0;-Tile_z/2], OP2=[0;0;Tile_z/2], OP3=[0;0;Tile_z/2], OP4=[0;0;0], OP5=[0;0;0]}
      mask prompts: m "Mass (Kg)"; Ig "Inertia (at G, Kg m^2)"; OG "OG (3x1 vector, m)"; n "Number of ports"; OP1 "OP1 (3x1 vector, m)"; OP2 "OP2 (3x1 vector, m)"; OP3 "OP3 (3x1 vector, m)"; OP4 "OP4 (3x1 vector, m)"; OP5 "OP5 (3x1 vector,m)"
      mask help:
      | 18nx6n dynamic model of a rigid body at n given points (ports) between wrenches applied at the n points (input) and the motions vectors at these points (output).
      |
      | 0: the reference point
      | G: the center of mass
      | Pi (i=1:n): the n given connection points (n<6).
      |
      | All parameters are expressed in the body frame.
      | Each parameter can be an uncertain parameter declared with "ureal"
      mask init:
      | MultiPortRigidFreeBody
      mask Help: web('Docmultiportrigidbase.html','-browser','-browser')
      mask TypeOptions n: 1 | 2 | 3 | 4 | 5
      mask DialogControl ParameterGroupVar Prompt: Main parameters
      mask DialogControl port1 Prompt: Port #1
      mask DialogControl port2 Prompt: #2
      mask DialogControl port3 Prompt: #3
      mask DialogControl port4 Prompt: #4
      mask DialogControl port5 Prompt: #5
      mask Display:
      | disp('Multi-port\n rigid free body\n (18nx6n)')
      | for ii=1:n
      |     port_label('input', ii,['W_{./body,P',num2str(ii),'}'],'interpreter','tex')
      |     port_label('output',ii,['m_{P',num2str(ii),'}'],'interpreter','tex')
      | end
  Variant Subsystem : Subsystem  Variant=on
  W_Container : Outport
  W_Endpoint : Outport  Port=2
  W_EE : Outport  Port=3
  wires:
  Tile/1(m_P1) -> Variant Subsystem/3(m_T1)
  Variant Subsystem/3(W_T1) -> Tile/1(W_./body,P1)
  Variant Subsystem/1(W_A) -> W_Endpoint/1
  m_Endpoint/1 -> Variant Subsystem/1(m_A)
  m_Container/1 -> Variant Subsystem/2(m_C)
  Variant Subsystem/2(W_C) -> W_Container/1
  m_EE/1 -> Variant Subsystem/4(m_EE)
  Variant Subsystem/4(W_EE) -> W_EE/1
  Tile/2(m_P2) -> 18x18 DCM/1
  18x18 DCM/1 -> Variant Subsystem/5(m_T2)
  6x6 DCM/1 -> Tile/2(W_./body,P2)
  Variant Subsystem/5(W_T2) -> 6x6 DCM/1

== system SDT_Control_Tuning/Dynamics/Tiles/Tile2 ==
  m_Container : Inport
  m_Endpoint : Inport  Port=2
  m_EE : Inport  Port=3
  18x18 DCM : SDTlibV1/3//6//18 DCM/18x18 DCM  rot=[0 1 0; 1 0 0; 0 0 -1]  transp=on
      settings: SourceProductName=SDTlib
  6x6 DCM : SDTlibV1/3//6//18 DCM/6x6 DCM  rot=[0 1 0; 1 0 0; 0 0 -1]  transp=off
      settings: SourceProductName=SDTlib
  Tile : Subsystem  mask(Multi-port rigid body (18nx6n)){m=m_T, Ig=J_T_T, OG=[0;0;0], n=2, OP1=[0;0;-Tile_z/2], OP2=[0;0;Tile_z/2], OP3=[0;0;Tile_z/2], OP4=[0;0;0], OP5=[0;0;0]}
      mask prompts: m "Mass (Kg)"; Ig "Inertia (at G, Kg m^2)"; OG "OG (3x1 vector, m)"; n "Number of ports"; OP1 "OP1 (3x1 vector, m)"; OP2 "OP2 (3x1 vector, m)"; OP3 "OP3 (3x1 vector, m)"; OP4 "OP4 (3x1 vector, m)"; OP5 "OP5 (3x1 vector,m)"
      mask help:
      | 18nx6n dynamic model of a rigid body at n given points (ports) between wrenches applied at the n points (input) and the motions vectors at these points (output).
      |
      | 0: the reference point
      | G: the center of mass
      | Pi (i=1:n): the n given connection points (n<6).
      |
      | All parameters are expressed in the body frame.
      | Each parameter can be an uncertain parameter declared with "ureal"
      mask init:
      | MultiPortRigidFreeBody
      mask Help: web('Docmultiportrigidbase.html','-browser','-browser')
      mask TypeOptions n: 1 | 2 | 3 | 4 | 5
      mask DialogControl ParameterGroupVar Prompt: Main parameters
      mask DialogControl port1 Prompt: Port #1
      mask DialogControl port2 Prompt: #2
      mask DialogControl port3 Prompt: #3
      mask DialogControl port4 Prompt: #4
      mask DialogControl port5 Prompt: #5
      mask Display:
      | disp('Multi-port\n rigid free body\n (18nx6n)')
      | for ii=1:n
      |     port_label('input', ii,['W_{./body,P',num2str(ii),'}'],'interpreter','tex')
      |     port_label('output',ii,['m_{P',num2str(ii),'}'],'interpreter','tex')
      | end
  Variant Subsystem : Subsystem  Variant=on
  W_Container : Outport
  W_Endpoint : Outport  Port=2
  W_EE : Outport  Port=3
  wires:
  Variant Subsystem/5(W_T2) -> 6x6 DCM/1
  6x6 DCM/1 -> Tile/2(W_./body,P2)
  18x18 DCM/1 -> Variant Subsystem/5(m_T2)
  Tile/2(m_P2) -> 18x18 DCM/1
  Variant Subsystem/4(W_EE) -> W_EE/1
  m_EE/1 -> Variant Subsystem/4(m_EE)
  Variant Subsystem/2(W_C) -> W_Container/1
  m_Container/1 -> Variant Subsystem/2(m_C)
  m_Endpoint/1 -> Variant Subsystem/1(m_A)
  Variant Subsystem/1(W_A) -> W_Endpoint/1
  Variant Subsystem/3(W_T1) -> Tile/1(W_./body,P1)
  Tile/1(m_P1) -> Variant Subsystem/3(m_T1)
